simulink model "Simple_App"  (R2024b)
settings: Solver=VariableStepAuto  StartTime=0.0  StopTime=10.0  MaxStep=0.000001  RelTol=1e-3
libraries: simulink x1
settings Model: Creator=abdal  LastModifiedBy=abdal

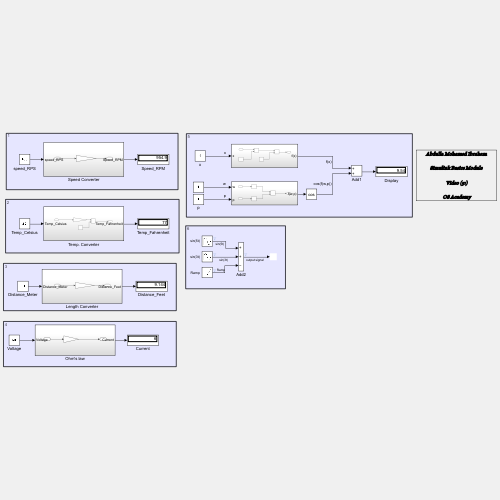
[thumbnail: Simulink's stored preview of the top-level diagram]
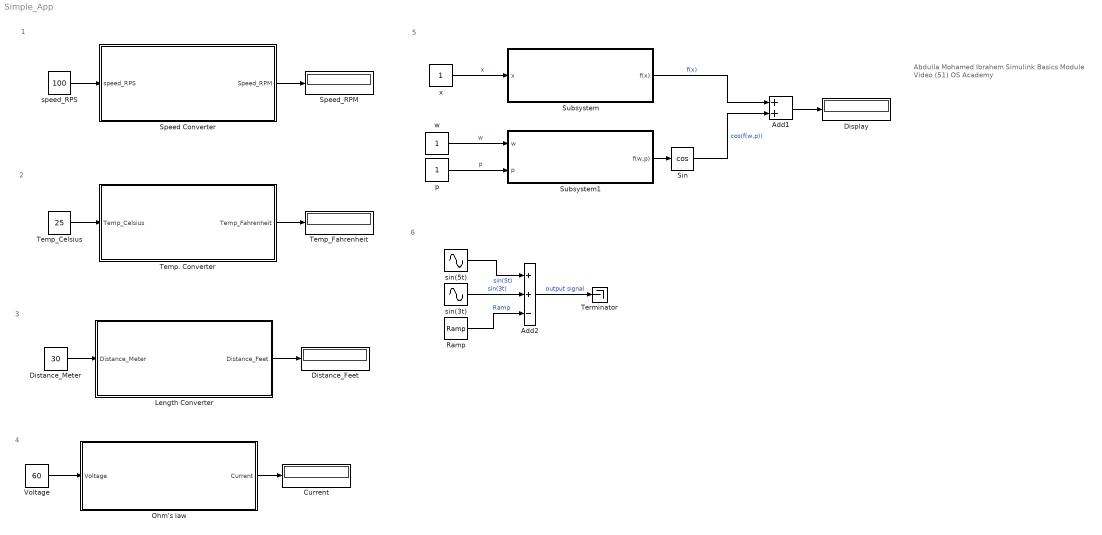
== system Simple_App ==
  note: 5
  note: 6
  note: 4
  note: 3
  note: 2
  note: 1
  note: Abdulla Mohamed Ibrahem
      | Simulink Basics Module
      | Video (51)
      | OS Academy
  Add1 : Sum
  Add2 : Sum  Inputs=++-
  Current : Display
  Display : Display
  Distance_Feet : Display
  Distance_Meter : Constant  Value=30
  Length Converter : Subsystem
  Ohm's law : Subsystem
  Ramp : simulink/Sources/Ramp  slope=1  start=0  InitialOutput=0
  Sin : Trigonometry  Operator=cos
  Speed Converter : Subsystem
  Speed_RPM : Display
  Subsystem : Subsystem
  Subsystem1 : Subsystem
  Temp. Converter : Subsystem
  Temp_Celsius : Constant  Value=25
  Temp_Fahrenheit : Display
  Terminator : Terminator
  Voltage : Constant  Value=60
  p : Constant
  sin(3t) : Sin  Frequency=3  SampleTime=0
  sin(5t) : Sin  Frequency=5  SampleTime=0
  speed_RPS : Constant  Value=100
  w : Constant
  x : Constant
  wires:
  speed_RPS/1 -> Speed Converter/1(speed_RPS)
  Speed Converter/1(Speed_RPM) -> Speed_RPM/1
  Temp_Celsius/1 -> Temp. Converter/1("Temp_Celsius ")
  Temp. Converter/1(Temp_Fahrenheit) -> Temp_Fahrenheit/1
  Length Converter/1(Distance_Feet) -> Distance_Feet/1
  Distance_Meter/1 -> Length Converter/1(Distance_Meter)
  Voltage/1 -> Ohm's law/1(Voltage)
  Ohm's law/1(Current) -> Current/1
  Sin/1 -> Add1/2  "cos(f(w,p))"
  Add1/1 -> Display/1
  x/1 -> Subsystem/1(x)  "x"
  Subsystem/1(f(x)) -> Add1/1  "f(x)"
  w/1 -> Subsystem1/1(w)  "w"
  p/1 -> Subsystem1/2(p)  "p"
  Subsystem1/1(f(w,p)) -> Sin/1
  sin(5t)/1 -> Add2/1  "sin(5t)"
  sin(3t)/1 -> Add2/2  "sin(3t)"
  Ramp/1 -> Add2/3  "Ramp"
  Add2/1 -> Terminator/1  "output signal"

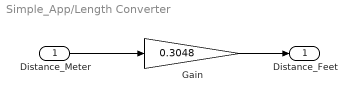
== system Simple_App/Length Converter ==
  Distance_Meter : Inport
  Gain : Gain  Gain=0.3048
  Distance_Feet : Outport
  wires:
  Gain/1 -> Distance_Feet/1
  Distance_Meter/1 -> Gain/1

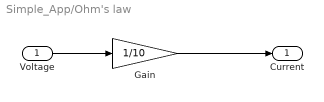
== system Simple_App/Ohm's law ==
  Voltage : Inport
  Gain : Gain  Gain=1/10
  Current : Outport
  wires:
  Voltage/1 -> Gain/1
  Gain/1 -> Current/1

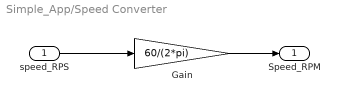
== system Simple_App/Speed Converter ==
  speed_RPS : Inport
  Gain : Gain  Gain=60/(2*pi)
  Speed_RPM : Outport
  wires:
  speed_RPS/1 -> Gain/1
  Gain/1 -> Speed_RPM/1

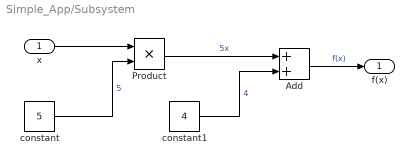
== system Simple_App/Subsystem ==
  x : Inport
  Add : Sum
  Product : Product
  constant : Constant  Value=5
  constant1 : Constant  Value=4
  f(x) : Outport
  wires:
  constant/1 -> Product/2  "5"
  constant1/1 -> Add/2  "4"
  Product/1 -> Add/1  "5x"
  Add/1 -> f(x)/1  "f(x)"
  x/1 -> Product/1

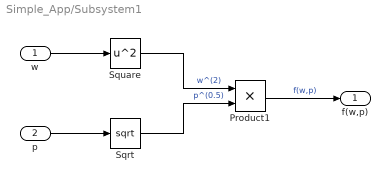
== system Simple_App/Subsystem1 ==
  w : Inport
  p : Inport  Port=2
  Product1 : Product
  Sqrt : Sqrt
  Square : Math  Operator=square
  f(w,p) : Outport
  wires:
  Square/1 -> Product1/1  "w^(2)"
  p/1 -> Sqrt/1
  w/1 -> Square/1
  Sqrt/1 -> Product1/2  "p^(0.5)"
  Product1/1 -> f(w,p)/1  "f(w,p)"

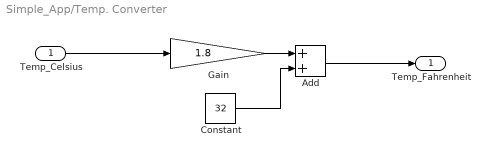
== system Simple_App/Temp. Converter ==
  "Temp_Celsius " : Inport
  Add : Sum
  Constant : Constant  Value=32
  Gain : Gain  Gain=1.8
  Temp_Fahrenheit : Outport
  wires:
  "Temp_Celsius "/1 -> Gain/1
  Gain/1 -> Add/1
  Constant/1 -> Add/2
  Add/1 -> Temp_Fahrenheit/1
